simulink model "D3D4"  (R2017b)
settings: Solver=VariableStepAuto  StartTime=0.0  StopTime=700  RelTol=1e-3
libraries: simulink x2, dspstat3 x1
settings Model: Creator=frank  LastModifiedBy=frank
settings SolverCC: ZeroCrossAlgorithm=Adaptive

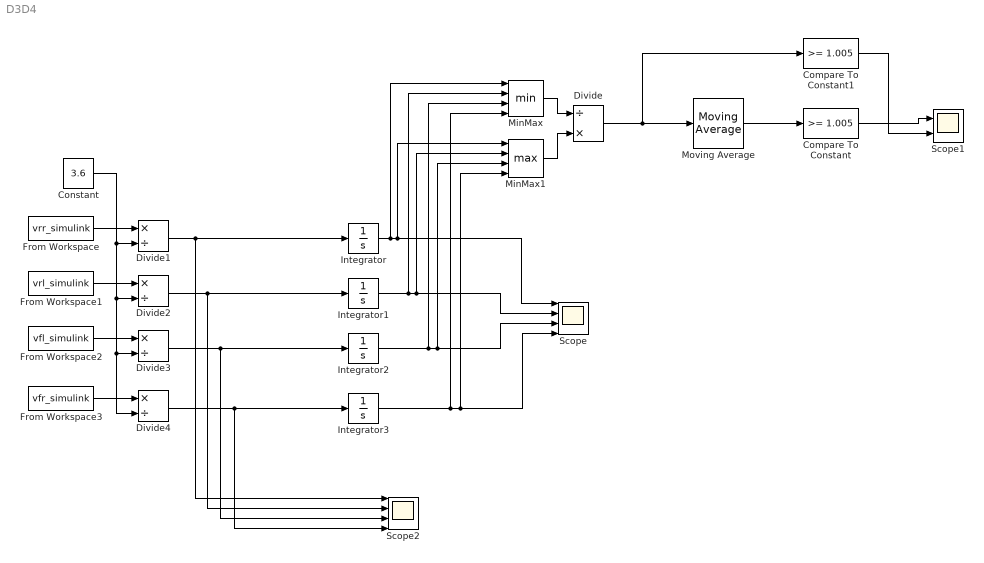
== system D3D4 ==
  Compare To Constant : simulink/Logic and Bit Operations/Compare To Constant  relop=>=  const=1.005  OutDataTypeStr=boolean
  Compare To Constant1 : simulink/Logic and Bit Operations/Compare To Constant  relop=>=  const=1.005  OutDataTypeStr=boolean
  Constant : Constant  Value=3.6
  Divide : Product  Inputs=/*
  Divide{1..4} (4 alike) : Product  Inputs=*/
  From Workspace : FromWorkspace  VariableName=vrr_simulink  SampleTime=0
  From Workspace1 : FromWorkspace  VariableName=vrl_simulink  SampleTime=0
  From Workspace2 : FromWorkspace  VariableName=vfl_simulink  SampleTime=0
  From Workspace3 : FromWorkspace  VariableName=vfr_simulink  SampleTime=0
  Integrator{,1..3} (4 alike) : Integrator
  MinMax : MinMax  Inputs=4
  MinMax1 : MinMax  Function=max  Inputs=4
  Moving Average : dspstat3/Moving Average  Method=Sliding window  SpecifyWindowLength=on  WindowLength=10  ForgettingFactor=0.9  SimulateUsing=Code generation
  Scope : Scope  NumInputPorts=4
  Scope1 : Scope  NumInputPorts=2
  Scope2 : Scope  NumInputPorts=4
  wires:
  Integrator/1 -> MinMax/1, MinMax1/1, Scope/1
  Integrator1/1 -> MinMax/2, MinMax1/2, Scope/2
  Integrator3/1 -> MinMax/4, MinMax1/4, Scope/4
  Integrator2/1 -> MinMax/3, MinMax1/3, Scope/3
  MinMax/1 -> Divide/1
  MinMax1/1 -> Divide/2
  Compare To Constant/1 -> Scope1/1
  Divide/1 -> Compare To Constant1/1, Moving Average/1
  Moving Average/1 -> Compare To Constant/1
  Compare To Constant1/1 -> Scope1/2
  From Workspace/1 -> Divide1/1
  Divide1/1 -> Scope2/1, Integrator/1
  From Workspace1/1 -> Divide2/1
  Divide2/1 -> Scope2/2, Integrator1/1
  From Workspace2/1 -> Divide3/1
  Divide3/1 -> Scope2/3, Integrator2/1
  From Workspace3/1 -> Divide4/1
  Divide4/1 -> Scope2/4, Integrator3/1
  Constant/1 -> Divide4/2, Divide3/2, Divide2/2, Divide1/2
